simulink model "BMSV001"  (R2025b)
settings: Solver=ode4  StartTime=0.0  StopTime=inf  FixedStep=0.005  RelTol=1e-3
settings Model: Creator=arull  LastModifiedBy=arull
settings DataIOCC: SaveOutput=off  SignalLogging=off  DSMLogging=off  SaveTime=off  ReturnWorkspaceOutputs=off
settings OptimizationCC: BlockReduction=off  DefaultParameterBehavior=Inlined  EnhancedBackFolding=on  PassReuseOutputArgsAs=Individual arguments  ZeroExternalMemoryAtStartup=off  ZeroInternalMemoryAtStartup=off  OptimizeBlockOrder=speed  DifferentSizesBufferReuse=on  OptimizationCustomize=off  EfficientTunableParamExpr=on
settings DebuggingCC: ParameterTunabilityLossMsg=error
settings HardwareCC: ProdBitPerPointer=32.0  ProdBitPerSizeT=32.0  ProdBitPerPtrDiffT=32.0  ProdLargestAtomicFloat=None  ProdWordSize=32.0  ProdHWDeviceType=Renesas->RH850
settings SFSimCC: MATLABDynamicMemAlloc=off
settings RTWCC: SystemTargetFile=ert.tlc  GenCodeOnly=on  TemplateMakefile=ert_default_tmf  Description=Embedded Coder
settings CodeAppCC: ForceParamTrailComments=on  IgnoreCustomStorageClasses=off  OperatorAnnotations=on  SimulinkDataObjDesc=on  SFDataObjDesc=on  InsertBlockDesc=on
settings ERTTargetCC: RTWCAPISignals=on  RTWCAPIRootIO=on  ERTCustomFileTemplate=example_file_process.tlc  TargetLangStandard=C99 (ISO)  GenerateSampleERTMain=on  SupportContinuousTime=on

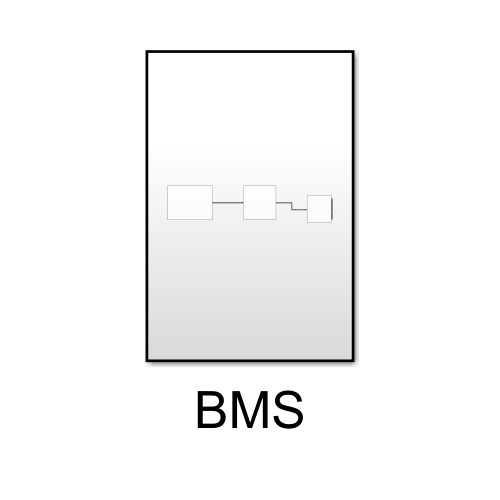
[thumbnail: Simulink's stored preview of the top-level diagram]
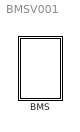
== system BMSV001 ==
  BMS : Subsystem

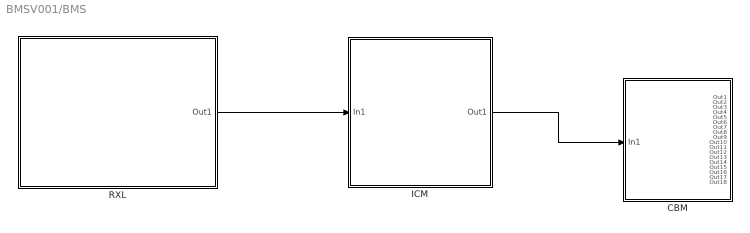
== system BMSV001/BMS ==
  CBM : Subsystem
  ICM : Subsystem
  RXL : Subsystem
  wires:
  RXL/1(Out1) -> ICM/1(In1)
  ICM/1(Out1) -> CBM/1(In1)

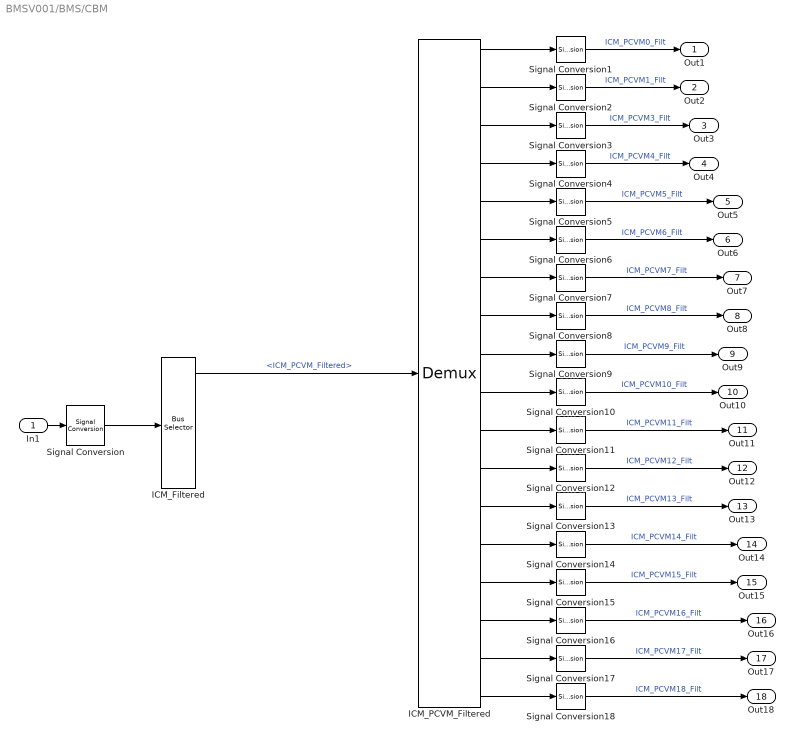
== system BMSV001/BMS/CBM ==
  In1 : Inport
  ICM_Filtered : BusSelector  OutputSignals=ICM_PCVM_Filtered,ICM_BVM_Filtered,ICM_AVM_Filtered,ICM_TEMPERATURE_Filtered
  ICM_PCVM_Filtered : Demux  Outputs=18
  Signal Conversion : SignalConversion  OverrideOpt=on
  Signal Conversion{1..18} (18 alike) : SignalConversion  OverrideOpt=off
  Out1 : Outport
  Out2 : Outport  Port=2
  Out3 : Outport  Port=3
  Out4 : Outport  Port=4
  Out5 : Outport  Port=5
  Out6 : Outport  Port=6
  Out7 : Outport  Port=7
  Out8 : Outport  Port=8
  Out9 : Outport  Port=9
  Out10 : Outport  Port=10
  Out11 : Outport  Port=11
  Out12 : Outport  Port=12
  Out13 : Outport  Port=13
  Out14 : Outport  Port=14
  Out15 : Outport  Port=15
  Out16 : Outport  Port=16
  Out17 : Outport  Port=17
  Out18 : Outport  Port=18
  wires:
  In1/1 -> Signal Conversion/1
  Signal Conversion/1 -> ICM_Filtered/1
  ICM_Filtered/1 -> ICM_PCVM_Filtered/1  "<ICM_PCVM_Filtered>"
  ICM_PCVM_Filtered/1 -> Signal Conversion1/1
  ICM_PCVM_Filtered/2 -> Signal Conversion2/1
  Signal Conversion1/1 -> Out1/1  "ICM_PCVM0_Filt"
  Signal Conversion2/1 -> Out2/1  "ICM_PCVM1_Filt"
  ICM_PCVM_Filtered/3 -> Signal Conversion3/1
  ICM_PCVM_Filtered/4 -> Signal Conversion4/1
  ICM_PCVM_Filtered/5 -> Signal Conversion5/1
  ICM_PCVM_Filtered/6 -> Signal Conversion6/1
  ICM_PCVM_Filtered/7 -> Signal Conversion7/1
  ICM_PCVM_Filtered/8 -> Signal Conversion8/1
  ICM_PCVM_Filtered/9 -> Signal Conversion9/1
  ICM_PCVM_Filtered/10 -> Signal Conversion10/1
  ICM_PCVM_Filtered/11 -> Signal Conversion11/1
  ICM_PCVM_Filtered/12 -> Signal Conversion12/1
  ICM_PCVM_Filtered/13 -> Signal Conversion13/1
  ICM_PCVM_Filtered/16 -> Signal Conversion16/1
  ICM_PCVM_Filtered/15 -> Signal Conversion15/1
  ICM_PCVM_Filtered/14 -> Signal Conversion14/1
  ICM_PCVM_Filtered/17 -> Signal Conversion17/1
  ICM_PCVM_Filtered/18 -> Signal Conversion18/1
  Signal Conversion4/1 -> Out4/1  "ICM_PCVM4_Filt"
  Signal Conversion3/1 -> Out3/1  "ICM_PCVM3_Filt"
  Signal Conversion7/1 -> Out7/1  "ICM_PCVM7_Filt"
  Signal Conversion8/1 -> Out8/1  "ICM_PCVM8_Filt"
  Signal Conversion6/1 -> Out6/1  "ICM_PCVM6_Filt"
  Signal Conversion5/1 -> Out5/1  "ICM_PCVM5_Filt"
  Signal Conversion9/1 -> Out9/1  "ICM_PCVM9_Filt"
  Signal Conversion10/1 -> Out10/1  "ICM_PCVM10_Filt"
  Signal Conversion12/1 -> Out12/1  "ICM_PCVM12_Filt"
  Signal Conversion11/1 -> Out11/1  "ICM_PCVM11_Filt"
  Signal Conversion14/1 -> Out14/1  "ICM_PCVM14_Filt"
  Signal Conversion15/1 -> Out15/1  "ICM_PCVM15_Filt"
  Signal Conversion13/1 -> Out13/1  "ICM_PCVM13_Filt"
  Signal Conversion17/1 -> Out17/1  "ICM_PCVM17_Filt"
  Signal Conversion16/1 -> Out16/1  "ICM_PCVM16_Filt"
  Signal Conversion18/1 -> Out18/1  "ICM_PCVM18_Filt"

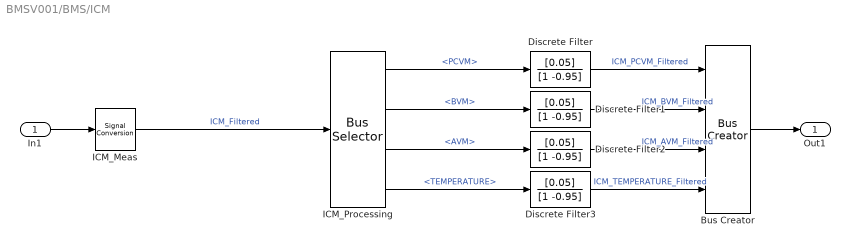
== system BMSV001/BMS/ICM ==
  In1 : Inport
  Bus Creator : BusCreator  Inputs=4
  Discrete Filter{,1..3} (4 alike) : DiscreteFilter  Numerator=[0.05]  Denominator=[1 -0.95]  a0EqualsOne=on
  ICM_Meas : SignalConversion  OverrideOpt=on
  ICM_Processing : BusSelector  OutputSignals=PCVM,BVM,AVM,TEMPERATURE
  Out1 : Outport
  wires:
  In1/1 -> ICM_Meas/1
  ICM_Meas/1 -> ICM_Processing/1  "ICM_Filtered"
  ICM_Processing/1 -> Discrete Filter/1  "<PCVM>"
  ICM_Processing/2 -> Discrete Filter1/1  "<BVM>"
  ICM_Processing/3 -> Discrete Filter2/1  "<AVM>"
  ICM_Processing/4 -> Discrete Filter3/1  "<TEMPERATURE>"
  Discrete Filter/1 -> Bus Creator/1  "ICM_PCVM_Filtered"
  Discrete Filter1/1 -> Bus Creator/2  "ICM_BVM_Filtered"
  Discrete Filter2/1 -> Bus Creator/3  "ICM_AVM_Filtered"
  Discrete Filter3/1 -> Bus Creator/4  "ICM_TEMPERATURE_Filtered"
  Bus Creator/1 -> Out1/1

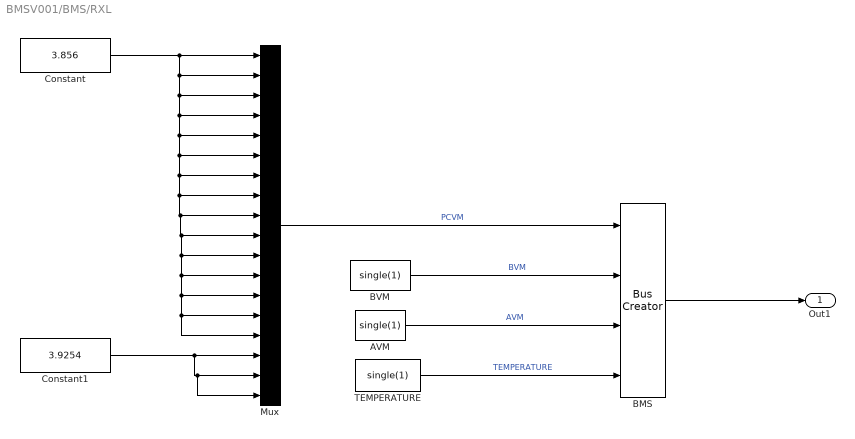
== system BMSV001/BMS/RXL ==
  AVM : Constant  Value=single(1)  OutDataTypeStr=single
  BMS : BusCreator  Inputs=4  OutDataTypeStr=Bus: Rxl_BMS  NonVirtualBus=on
  BVM : Constant  Value=single(1)  OutDataTypeStr=single
  Constant : Constant  Value=3.856  OutDataTypeStr=single
  Constant1 : Constant  Value=3.9254  OutDataTypeStr=single
  Mux : Mux  Inputs=18
  TEMPERATURE : Constant  Value=single(1)  OutDataTypeStr=single
  Out1 : Outport
  wires:
  Mux/1 -> BMS/1  "PCVM"
  TEMPERATURE/1 -> BMS/4  "TEMPERATURE"
  BVM/1 -> BMS/2  "BVM"
  AVM/1 -> BMS/3  "AVM"
  BMS/1 -> Out1/1
  Constant/1 -> Mux/15, Mux/14, Mux/13, Mux/12, Mux/11, Mux/10, Mux/9, Mux/8, Mux/7, Mux/6, Mux/5, Mux/4, Mux/3, Mux/2, Mux/1
  Constant1/1 -> Mux/18, Mux/17, Mux/16
